simulink model "lab5_ASP_GejsisD"  (R2018b)
settings: Solver=VariableStepAuto  StartTime=0.0  StopTime=10.0  RelTol=1e-3
libraries: dspsrcs4 x2, dspsnks4 x1, dspvision x1
settings Model: Creator=Student  LastModifiedBy=Student

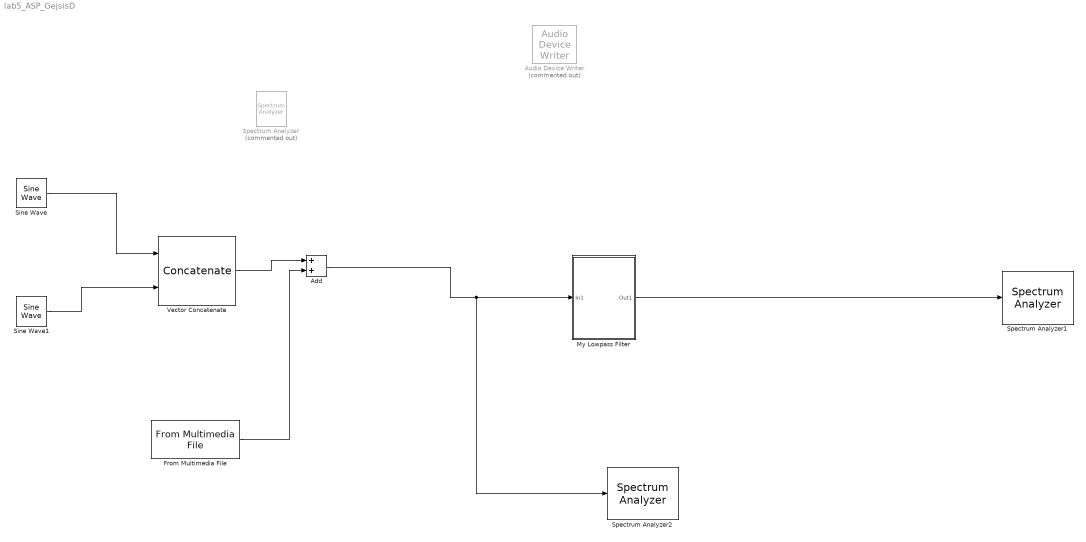
== system lab5_ASP_GejsisD ==
  Add : Sum
  Audio Device Writer : dspsnks4/Audio Device Writer  Commented=on  Driver=DirectSound  Device=Default  InheritSampleRate=on  SampleRate=44100  BitDepth=16-bit integer  BufferSize=4096  NumBuffers=10  DefaultOutputChannelMapping=on  OutputChannelMapping=1:2  OutputNumUnderrunSamples=off  DriverIdx=1  DeviceWarnFlag=''
  From Multimedia File : dspvision/From Multimedia File  inputFilename=song.mp3  loop=on  numPlays=inf  outputStreams=Audio only  videoDataType=single  audioDataType=double  inheritSampleTime=on  userDefinedSampleTime=1/30  noAudioOutput=off  isIntensityVideo=off  fourcc=RGB  colorVideoFormat=Separate color signals  outputEOF=off  dataOrg=Column-major  audioFrameSize=1024  computeAudioFrameSize=off  outSamplingMode=Sample based
      settings: SourceProductBaseCode=VP
  My Lowpass Filter : Subsystem
  Sine Wave : dspsrcs4/Sine Wave  Amplitude=1  Frequency=17000  Phase=0  SampleMode=Discrete  OutComplex=Real  CompMethod=Trigonometric fcn  TableSize=Speed  SampleTime=1/44100  SamplesPerFrame=1024  ResetState=Restart at time zero  OutputFrames=off  dataType=double  wordLen=16  udDataType=sfix(16)  fracBitsMode=Best precision  numFracBits=15  OutDataTypeStr=double  LastOutDataTypeStr=double
  Sine Wave1 : dspsrcs4/Sine Wave  Amplitude=1  Frequency=17000  Phase=0  SampleMode=Discrete  OutComplex=Real  CompMethod=Trigonometric fcn  TableSize=Speed  SampleTime=1/44100  SamplesPerFrame=1024  ResetState=Restart at time zero  OutputFrames=off  dataType=double  wordLen=16  udDataType=sfix(16)  fracBitsMode=Best precision  numFracBits=15  OutDataTypeStr=double  LastOutDataTypeStr=double
  Spectrum Analyzer : SpectrumAnalyzer  Commented=on
  Spectrum Analyzer1 : SpectrumAnalyzer
  Spectrum Analyzer2 : SpectrumAnalyzer
  Vector Concatenate : Concatenate  Mode=Multidimensional array  ConcatenateDimension=2
  wires:
  Sine Wave/1 -> Vector Concatenate/1
  Sine Wave1/1 -> Vector Concatenate/2
  My Lowpass Filter/1(Out1) -> Spectrum Analyzer1/1
  Add/1 -> Spectrum Analyzer2/1, My Lowpass Filter/1(In1)
  Vector Concatenate/1 -> Add/1
  From Multimedia File/1 -> Add/2

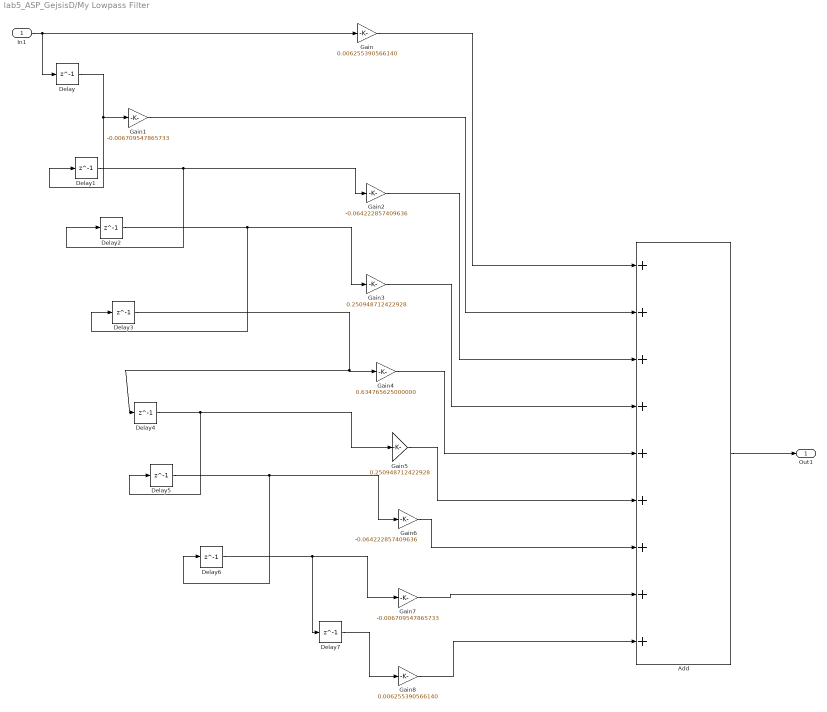
== system lab5_ASP_GejsisD/My Lowpass Filter ==
  In1 : Inport
  Add : Sum  Inputs=+++++++++
  Delay{,1..7} (8 alike) : Delay  DelayLength=1  InitialCondition=0
  Gain : Gain  Gain=0.006255390566140
  Gain1 : Gain  Gain=-0.006709547865733
  Gain2 : Gain  Gain=-0.064222857409636
  Gain3 : Gain  Gain=0.250948712422928
  Gain4 : Gain  Gain=0.634765625000000
  Gain5 : Gain  Gain=0.250948712422928
  Gain6 : Gain  Gain=-0.064222857409636
  Gain7 : Gain  Gain=-0.006709547865733
  Gain8 : Gain  Gain=0.006255390566140
  Out1 : Outport
  wires:
  In1/1 -> Delay/1, Gain/1
  Gain5/1 -> Add/6
  Delay7/1 -> Gain8/1
  Delay4/1 -> Delay5/1, Gain5/1
  Gain8/1 -> Add/9
  Gain3/1 -> Add/4
  Delay5/1 -> Delay6/1, Gain6/1
  Gain1/1 -> Add/2
  Gain7/1 -> Add/8
  Delay1/1 -> Delay2/1, Gain2/1
  Add/1 -> Out1/1
  Gain6/1 -> Add/7
  Gain4/1 -> Add/5
  Gain/1 -> Add/1
  Gain2/1 -> Add/3
  Delay2/1 -> Delay3/1, Gain3/1
  Delay3/1 -> Delay4/1, Gain4/1
  Delay/1 -> Delay1/1, Gain1/1
  Delay6/1 -> Delay7/1, Gain7/1
